simulink model "CVS_Model"  (R2023b)
settings: Solver=ode3  StartTime=0.0  StopTime=max(simulation_time)  FixedStep=0.01  RelTol=1e-3  EnableMultiTasking=on
values from neighbouring files (symbols this model uses):
  A1 = x(1)    [Cohort_Generation.m]
  A2 = x(2)    [Cohort_Generation.m]
  A3 = x(8)    [Cohort_Generation.m]
  A4 = x(12)    [Cohort_Generation.m]
  B_Gain = x(3)    [Cohort_Generation.m]
  B_Loss = x(4)    [Cohort_Generation.m]
  BP_Tar = x(14)    [Cohort_Generation.m]
  BV0 = BV0_aux+rand_IC*BV0_aux*randn    [Cohort_Generation.m]
  G1 = x(15)    [Cohort_Generation.m]
  G2 = x(16)    [Cohort_Generation.m]
  G3 = x(19)    [Cohort_Generation.m]
  Gsv1 = x(6)    [Cohort_Generation.m]
  Gsv2 = x(7)    [Cohort_Generation.m]
  Hct0 = Hct0_aux+rand_IC*Hct0_aux*randn    [Cohort_Generation.m]
  HR0 = Hemo_HR(1)+rand_IC*Hemo_HR(1)*randn    [Cohort_Generation.m]
  Ki4 = x(21)    [Cohort_Generation.m]
  Kp = x(5)    [Cohort_Generation.m]
  Kp2 = x(10)    [Cohort_Generation.m]
  Kp3 = x(11)    [Cohort_Generation.m]
  Kp4 = x(20)    [Cohort_Generation.m]
  pow1 = x(17)    [Cohort_Generation.m]
  pow2 = x(18)    [Cohort_Generation.m]
  SV0 = SV0_aux+rand_IC*SV0_aux*randn    [Cohort_Generation.m]
  SV_Tar = x(9)    [Cohort_Generation.m]
  TPR0 = (Hemo_MAP(1)/Hemo_CO(1))+rand_IC*(Hemo_MAP(1)/Hemo_CO(1))*randn    [Cohort_Generation.m]
libraries: simulink x7
settings Model: Creator=Ramin  LastModifiedBy=raminbighamian
settings SolverCC: AlgebraicLoopSolver=TrustRegion
settings DataIOCC: LimitDataPoints=on  SaveFormat=Array  SignalLoggingSaveFormat=ModelDataLogs  ReturnWorkspaceOutputs=off
settings OptimizationCC: ExpressionDepthLimit=2147483647  LifeSpan=inf
settings DebuggingCC: UnderspecifiedInitializationDetection=Classic  MergeDetectMultiDrivingBlocksExec=none  SolverPrmCheckMsg=warning  FcnCallInpInsideContextMsg=warning  UnconnectedInputMsg=warning  UnconnectedOutputMsg=warning  UnconnectedLineMsg=warning  StateNameClashWarn=warning  SFUnexpectedBacktrackingDiag=warning  SFNoUnconditionalDefaultTransitionDiag=warning  SFExecutionAtInitializationDiag=none  ArithmeticOperatorsInVariantConditions=warning
settings HardwareCC: ProdBitPerPointer=32  ProdBitPerSizeT=32  ProdBitPerPtrDiffT=32  ProdLargestAtomicFloat=None  ProdIntDivRoundTo=Undefined  ProdEndianess=Unspecified  ProdWordSize=32  ProdHWDeviceType=32-bit Generic
settings ModelReferenceCC: EnableRefExpFcnMdlSchedulingChecks=on  PropagateSignalLabelsOutOfModel=off
settings SFSimCC: SimUseLocalCustomCode=off  CustomCodeUndefinedFunction=UseInterfaceOnly
settings RTWCC: RTWUseLocalCustomCode=off
settings CodeAppCC: StateflowObjectComments=on
settings GRTTargetCC: TargetLangStandard=C89/C90 (ANSI)
settings ConfigComp: CovMetricSettings=dw  CovSaveCumulativeToWorkspaceVar=on  CovSaveSingleToWorkspaceVar=on  CovExternalEMLEnable=off

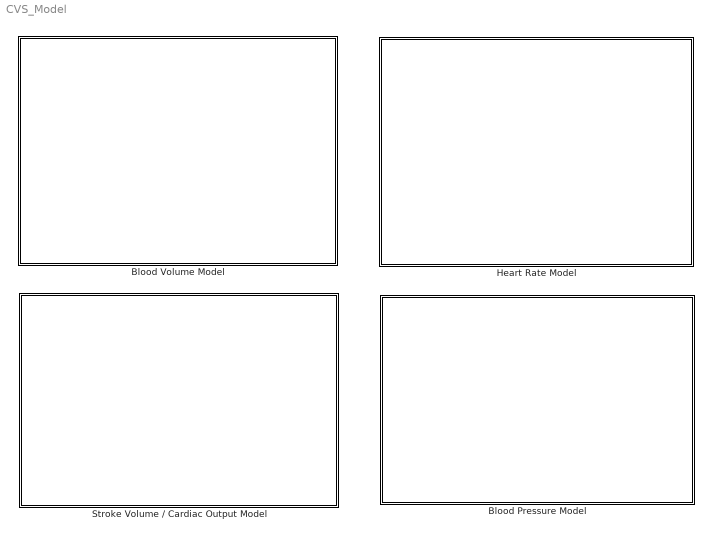
== system CVS_Model ==
  Blood Pressure Model : Subsystem
  Blood Volume Model : Subsystem
  Heart Rate Model : Subsystem
  Stroke Volume / Cardiac Output Model : Subsystem

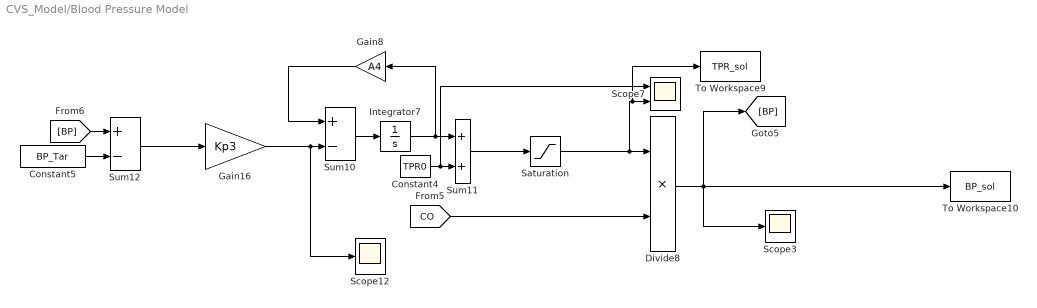
== system CVS_Model/Blood Pressure Model ==
  Constant4 : Constant  Value=TPR0
  Constant5 : Constant  Value=BP_Tar
  Divide8 : Product  Inputs=**
  Gain16 : Gain  Gain=Kp3
  Gain8 : Gain  Gain=A4
  Integrator7 : Integrator
  Saturation : Saturate  UpperLimit=4000  LowerLimit=0
  Scope12 : Scope
  Scope3 : Scope
  Scope7 : Scope  NumInputPorts=2
  Sum10 : Sum  Inputs=+-
  Sum11 : Sum
  Sum12 : Sum  Inputs=+-
  To Workspace10 : ToWorkspace  VariableName=BP_sol  SampleTime=-1
  To Workspace9 : ToWorkspace  VariableName=TPR_sol  SampleTime=-1
  wires:
  [BP] -> Sum12/1
  Sum10/1 -> Integrator7/1
  [CO] -> Divide8/2
  Saturation/1 -> To Workspace9/1, Scope7/2, Divide8/1
  Integrator7/1 -> Gain8/1, Sum11/1
  Constant5/1 -> Sum12/2
  Gain16/1 -> Scope12/1, Sum10/2
  Sum11/1 -> Saturation/1
  Gain8/1 -> Sum10/1
  Constant4/1 -> Scope7/1, Sum11/2
  Divide8/1 -> To Workspace10/1, Scope3/1, [BP]
  Sum12/1 -> Gain16/1

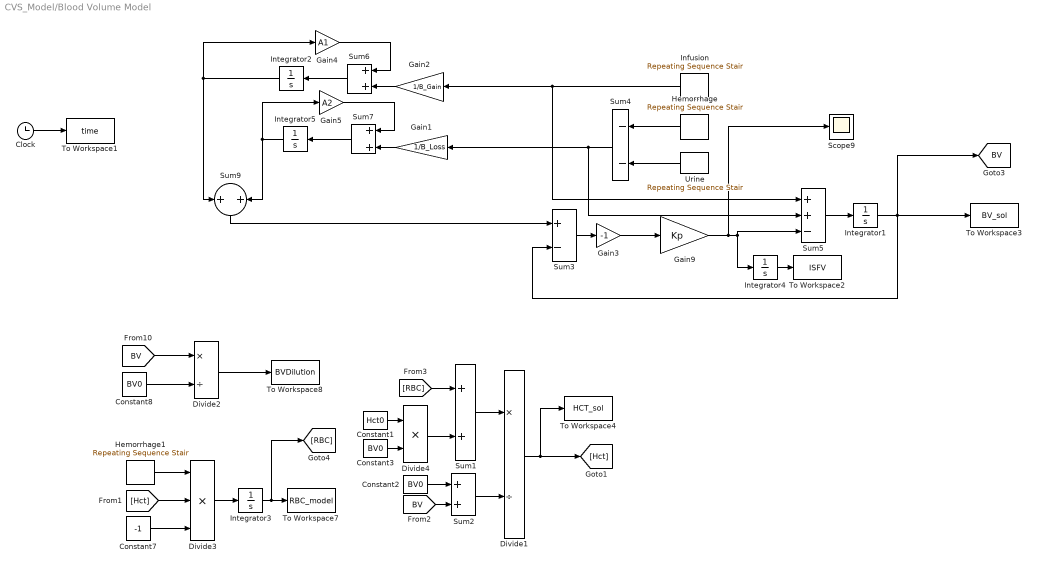
== system CVS_Model/Blood Volume Model ==
  Clock : Clock
  Constant1 : Constant  Value=Hct0
  Constant2 : Constant  Value=BV0
  Constant3 : Constant  Value=BV0
  Constant7 : Constant  Value=-1
  Constant8 : Constant  Value=BV0
  Divide1 : Product  Inputs=*/
  Divide2 : Product  Inputs=*/
  Divide3 : Product  Inputs=***
  Divide4 : Product  Inputs=**
  Gain1 : Gain  Gain=1/B_Loss
  Gain2 : Gain  Gain=1/B_Gain
  Gain3 : Gain  Gain=-1
  Gain4 : Gain  Gain=A1
  Gain5 : Gain  Gain=A2
  Gain9 : Gain  Gain=Kp
  Hemorrhage : simulink/Sources/Repeating Sequence Stair  OutValues=Hemorrhage_inp  tsamp=SamplingTime  OutMin=[]  OutMax=[]  OutDataTypeStr=double  OutputDataTypeScalingMode=double  OutDataType=fixdt(0,8)  ConRadixGroup=Best Precision: Vector-wise  OutScaling=2^-12
  Hemorrhage1 : simulink/Sources/Repeating Sequence Stair  OutValues=Hemorrhage_inp  tsamp=SamplingTime  OutMin=[]  OutMax=[]  OutDataTypeStr=double  OutputDataTypeScalingMode=double  OutDataType=fixdt(0,8)  ConRadixGroup=Best Precision: Vector-wise  OutScaling=2^-12
  Infusion : simulink/Sources/Repeating Sequence Stair  OutValues=Infusion_inp  tsamp=SamplingTime  OutMin=[]  OutMax=[]  OutDataTypeStr=double  OutputDataTypeScalingMode=double  OutDataType=fixdt(0,8)  ConRadixGroup=Best Precision: Vector-wise  OutScaling=2^-12
  Integrator{1..5} (5 alike) : Integrator
  Scope9 : Scope
  Sum{1..2,6..7,9} (5 alike) : Sum
  Sum3 : Sum  Inputs=+-
  Sum4 : Sum  Inputs=--
  Sum5 : Sum  Inputs=++-
  To Workspace1 : ToWorkspace  VariableName=time  SampleTime=-1
  To Workspace2 : ToWorkspace  VariableName=ISFV  SampleTime=-1
  To Workspace3 : ToWorkspace  VariableName=BV_sol  SampleTime=-1
  To Workspace4 : ToWorkspace  VariableName=HCT_sol  SampleTime=-1
  To Workspace7 : ToWorkspace  VariableName=RBC_model  SampleTime=-1
  To Workspace8 : ToWorkspace  VariableName=BVDilution  SampleTime=-1
  Urine : simulink/Sources/Repeating Sequence Stair  OutValues=Urine_inp  tsamp=SamplingTime  OutMin=[]  OutMax=[]  OutDataTypeStr=double  OutputDataTypeScalingMode=double  OutDataType=fixdt(0,8)  ConRadixGroup=Best Precision: Vector-wise  OutScaling=2^-12
  tag scope: BV=global
  wires:
  Sum3/1 -> Gain3/1
  Sum5/1 -> Integrator1/1
  Divide3/1 -> Integrator3/1
  Constant7/1 -> Divide3/3
  Sum6/1 -> Integrator2/1
  Gain5/1 -> Sum7/1
  Sum2/1 -> Divide1/2
  Gain9/1 -> Scope9/1, Sum5/3, Integrator4/1
  Divide2/1 -> To Workspace8/1
  Gain1/1 -> Sum7/2
  Gain2/1 -> Sum6/2
  Integrator5/1 -> Sum9/2, Gain5/1
  Gain4/1 -> Sum6/1
  Hemorrhage/1 -> Sum4/1
  [BV] -> Divide2/1
  Sum7/1 -> Integrator5/1
  Integrator1/1 -> Sum3/2, To Workspace3/1, [BV]
  Integrator3/1 -> [RBC], To Workspace7/1
  [RBC] -> Sum1/1
  Divide4/1 -> Sum1/2
  Integrator4/1 -> To Workspace2/1
  [Hct] -> Divide3/2
  Urine/1 -> Sum4/2
  Infusion/1 -> Sum5/1, Gain2/1
  [BV] -> Sum2/2
  Divide1/1 -> [Hct], To Workspace4/1
  Sum1/1 -> Divide1/1
  Hemorrhage1/1 -> Divide3/1
  Constant8/1 -> Divide2/2
  Constant2/1 -> Sum2/1
  Sum9/1 -> Sum3/1
  Constant1/1 -> Divide4/1
  Constant3/1 -> Divide4/2
  Gain3/1 -> Gain9/1
  Sum4/1 -> Gain1/1, Sum5/2
  Integrator2/1 -> Sum9/1, Gain4/1
  Clock/1 -> To Workspace1/1

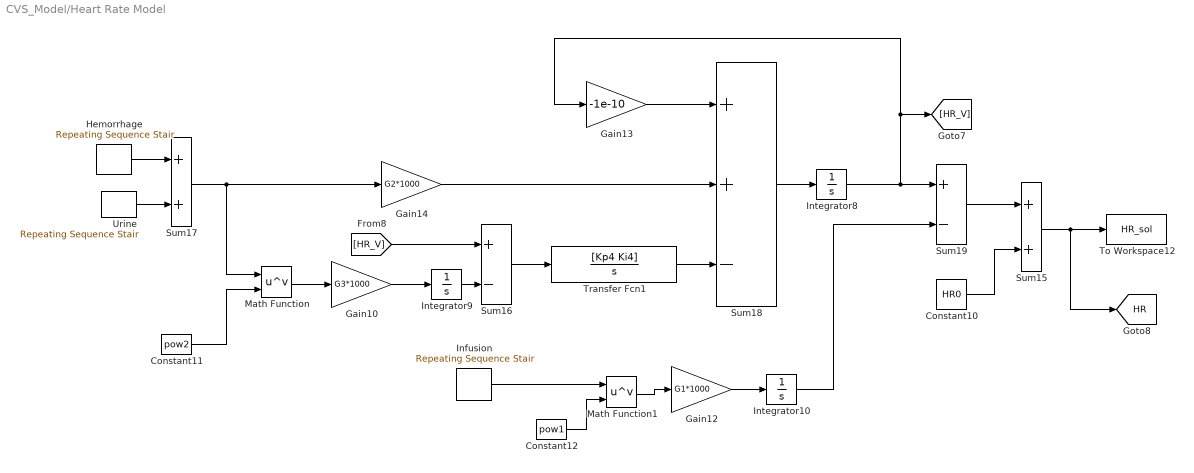
== system CVS_Model/Heart Rate Model ==
  Constant10 : Constant  Value=HR0
  Constant11 : Constant  Value=pow2
  Constant12 : Constant  Value=pow1
  Gain10 : Gain  Gain=G3*1000
  Gain12 : Gain  Gain=G1*1000
  Gain13 : Gain  Gain=-1e-10
  Gain14 : Gain  Gain=G2*1000
  Hemorrhage : simulink/Sources/Repeating Sequence Stair  OutValues=Hemorrhage_inp  tsamp=SamplingTime  OutMin=[]  OutMax=[]  OutDataTypeStr=double  OutputDataTypeScalingMode=double  OutDataType=fixdt(0,8)  ConRadixGroup=Best Precision: Vector-wise  OutScaling=2^-12
  Infusion : simulink/Sources/Repeating Sequence Stair  OutValues=Infusion_inp  tsamp=SamplingTime  OutMin=[]  OutMax=[]  OutDataTypeStr=double  OutputDataTypeScalingMode=double  OutDataType=fixdt(0,8)  ConRadixGroup=Best Precision: Vector-wise  OutScaling=2^-12
  Integrator10 : Integrator
  Integrator8 : Integrator
  Integrator9 : Integrator
  Math Function : Math  Operator=pow  SignedPower=on
  Math Function1 : Math  Operator=pow  SignedPower=on
  Sum15 : Sum
  Sum16 : Sum  Inputs=+-
  Sum17 : Sum
  Sum18 : Sum  Inputs=++-
  Sum19 : Sum  Inputs=+-
  To Workspace12 : ToWorkspace  VariableName=HR_sol  SampleTime=-1
  Transfer Fcn1 : TransferFcn  Numerator=[Kp4 Ki4]  Denominator=[1 0]
  Urine : simulink/Sources/Repeating Sequence Stair  OutValues=Urine_inp  tsamp=SamplingTime  OutMin=[]  OutMax=[]  OutDataTypeStr=double  OutputDataTypeScalingMode=double  OutDataType=fixdt(0,8)  ConRadixGroup=Best Precision: Vector-wise  OutScaling=2^-12
  tag scope: HR=global
  wires:
  Infusion/1 -> Math Function1/1
  Urine/1 -> Sum17/2
  Math Function1/1 -> Gain12/1
  Gain12/1 -> Integrator10/1
  [HR_V] -> Sum16/1
  Sum17/1 -> Gain14/1, Math Function/1
  Constant10/1 -> Sum15/2
  Integrator8/1 -> [HR_V], Gain13/1, Sum19/1
  Integrator10/1 -> Sum19/2
  Gain14/1 -> Sum18/2
  Constant11/1 -> Math Function/2
  Sum18/1 -> Integrator8/1
  Integrator9/1 -> Sum16/2
  Hemorrhage/1 -> Sum17/1
  Sum15/1 -> [HR], To Workspace12/1
  Gain10/1 -> Integrator9/1
  Transfer Fcn1/1 -> Sum18/3
  Gain13/1 -> Sum18/1
  Sum19/1 -> Sum15/1
  Math Function/1 -> Gain10/1
  Sum16/1 -> Transfer Fcn1/1
  Constant12/1 -> Math Function1/2

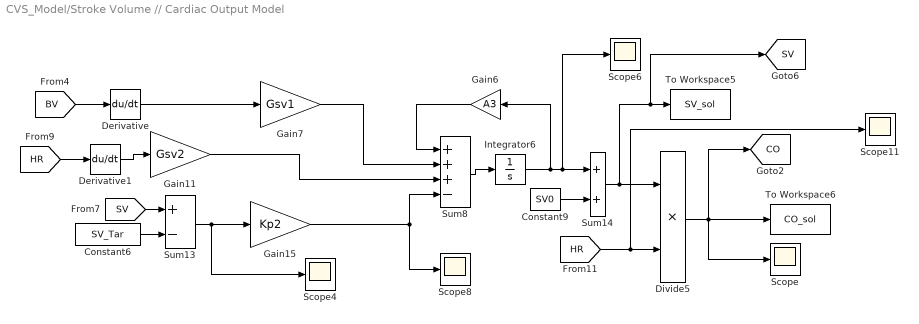
== system CVS_Model/Stroke Volume // Cardiac Output Model ==
  Constant6 : Constant  Value=SV_Tar
  Constant9 : Constant  Value=SV0
  Derivative : Derivative
  Derivative1 : Derivative
  Divide5 : Product  Inputs=**
  Gain11 : Gain  Gain=Gsv2
  Gain15 : Gain  Gain=Kp2
  Gain6 : Gain  Gain=A3
  Gain7 : Gain  Gain=Gsv1
  Integrator6 : Integrator
  Scope{,4,6,8,11} (5 alike) : Scope
  Sum13 : Sum  Inputs=+-
  Sum14 : Sum
  Sum8 : Sum  Inputs=+++-
  To Workspace5 : ToWorkspace  VariableName=SV_sol  SampleTime=-1
  To Workspace6 : ToWorkspace  VariableName=CO_sol  SampleTime=-1
  tag scope: CO=global, SV=global
  wires:
  Integrator6/1 -> Sum14/1, Scope6/1, Gain6/1
  Sum8/1 -> Integrator6/1
  Gain6/1 -> Sum8/1
  Derivative/1 -> Gain7/1
  Constant9/1 -> Sum14/2
  Gain7/1 -> Sum8/2
  Derivative1/1 -> Gain11/1
  Gain11/1 -> Sum8/3
  [SV] -> Sum13/1
  Divide5/1 -> [CO], To Workspace6/1, Scope/1
  Gain15/1 -> Scope8/1, Sum8/4
  [HR] -> Scope11/1, Divide5/2
  [HR] -> Derivative1/1
  Sum13/1 -> Gain15/1, Scope4/1
  [BV] -> Derivative/1
  Constant6/1 -> Sum13/2
  Sum14/1 -> [SV], To Workspace5/1, Divide5/1
